simulink model "OFDM_Tx_HW"  (R2020a)
settings: Solver=FixedStepDiscrete  StartTime=0.0  StopTime=inf  RelTol=1e-3
InitFcn:
  | % Set parameters
  | fs = 20e6;
  | fclk = 240e6;
  | ssr = 2;
  | fdc = fclk*ssr*8;
  | 
  | % Load libraries
  | addpath('./lib');
  | 
  | % Load all required variables
  | load('variables/read_addr_data');
  | load('variables/read_addr_cp');
  | load('variables/read_addr_pream');
  | load('variables/read_addr_rx');
  | load('variables/pilot');
  | load('variables/sc_index');
  | load('variables/LTSfreq');
  | load('variables/STSfreq');
  | load('variables/LTSread');
  | load('variables/STSread');
  | 
  | run ./scripts/rfgen;
undefined symbols (not defined in the file): LTSfreq, LTSread, pilot, read_addr_cp, read_addr_data, read_addr_pream, STSfreq, STSread
libraries: hdlsllib x28, simulink x15, lib_rfsignalgenerator x1, dsphdlxfrm x1, dspsigops x1
settings Model: DataTypeOverride=Off  Creator=njb13206  LastModifiedBy=andy
settings OptimizationCC: BlockReduction=off  ConditionallyExecuteInputs=off  DefaultParameterBehavior=Inlined
settings DebuggingCC: AlgebraicLoopMsg=error  SingleTaskRateTransMsg=error  IntegerOverflowMsg=none  ParameterPrecisionLossMsg=none  IntegerSaturationMsg=none
settings HardwareCC: ProdBitPerPointer=32  ProdBitPerSizeT=32  ProdBitPerPtrDiffT=32  ProdLargestAtomicFloat=None  ProdIntDivRoundTo=Undefined  ProdEndianess=Unspecified  ProdWordSize=32  ProdHWDeviceType=ASIC/FPGA->ASIC/FPGA  TargetBitPerLong=64  TargetBitPerPointer=64  TargetBitPerSizeT=64  TargetBitPerPtrDiffT=64  TargetLongLongMode=on  TargetIntDivRoundTo=Zero  TargetEndianess=LittleEndian  TargetWordSize=64  TargetHWDeviceType=Custom Processor->MATLAB Host Computer  ProdEqTarget=off

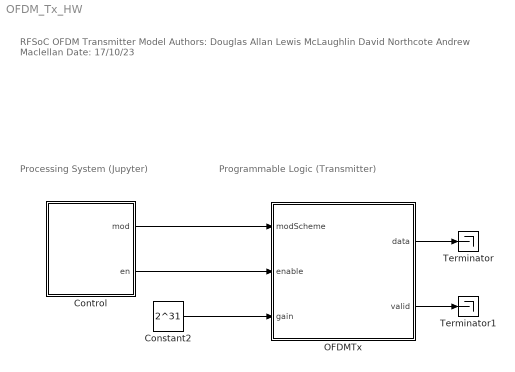
== system OFDM_Tx_HW ==
  note: RFSoC OFDM Transmitter Model
      | Authors: Douglas Allan
      | Lewis McLaughlin
      | David Northcote
      | Andrew Maclellan
      | Date: 17/10/23
  note: Programmable Logic (Transmitter)
  note: Processing System (Jupyter)
  Constant2 : Constant  Value=2^31  OutDataTypeStr=uint32  SampleTime=1/fclk
  Control : Subsystem  mask{mod_mask=128QAM, en=on}
      mask prompts: mod_mask "Modulation"; en "Enable"
      mask init:
      | % RF Signal Generator
      | if strcmpi(get_param(gcb, 'mod_mask'), 'BPSK')
      |     mod = 0;
      | elseif strcmpi(get_param(gcb, 'mod_mask'), 'QPSK')
      |     mod = 1;
      | elseif strcmpi(get_param(gcb, 'mod_mask'), '8PSK')
      |     mod = 2;
      | elseif strcmpi(get_param(gcb, 'mod_mask'), '16QAM')
      |     mod = 3;
      | elseif strcmpi(get_param(gcb, 'mod_mask'), '32QAM')
      |     mod = 4;
      | elseif strcmpi(get_param(gcb, 'mod_mask'), '64QAM')
      |     mod = 5;
      | elseif strcmpi(get_param(gcb, 'mod_mask'), '128QAM')
      |     mod = 6;
      | elseif strcmpi(get_param(gcb, 'mod_mask'), '256QAM')
      |     mod = 7;
      | elseif strcmpi(get_param(gcb, 'mod_mask'), '512QAM')
      |     mod = 8;
      | elseif strcmpi(get_param(gcb, 'mod_mask'), '1024QAM')
      |     mod = 9;
      | end
      mask TypeOptions mod_mask: BPSK | QPSK | 8PSK | 16QAM | 32QAM | 64QAM | 128QAM | 256QAM | 512QAM | 1024QAM
      mask DialogControl DescGroupVar Prompt: RF Signal Generator
      mask DialogControl DescTextVar Prompt: Exposes parameters the user can control from Jupyter when running on the target.
      mask DialogControl Container3 Prompt: Control
  OFDMTx : Subsystem  TreatAsAtomicUnit=on
  Terminator : Terminator
  Terminator1 : Terminator
  wires:
  Control/1(mod) -> OFDMTx/1(modScheme)
  Control/2(en) -> OFDMTx/2(enable)
  Constant2/1 -> OFDMTx/3(gain)
  OFDMTx/1(data) -> Terminator/1
  OFDMTx/2(valid) -> Terminator1/1

== system OFDM_Tx_HW/Control ==
  Constant2 : Constant  Value=en  OutDataTypeStr=boolean  SampleTime=1/(fclk)
  Constant7 : Constant  Value=mod  VectorParams1D=off  OutDataTypeStr=uint32  SampleTime=1/(fclk)
  Delay : Delay  DelayLength=randi(10)
  Delay3 : Delay  DelayLength=randi(10)
  mod : Outport  VectorParamsAs1DForOutWhenUnconnected=off
  en : Outport  Port=2  VectorParamsAs1DForOutWhenUnconnected=off
  wires:
  Constant2/1 -> Delay3/1
  Constant7/1 -> Delay/1
  Delay/1 -> mod/1
  Delay3/1 -> en/1

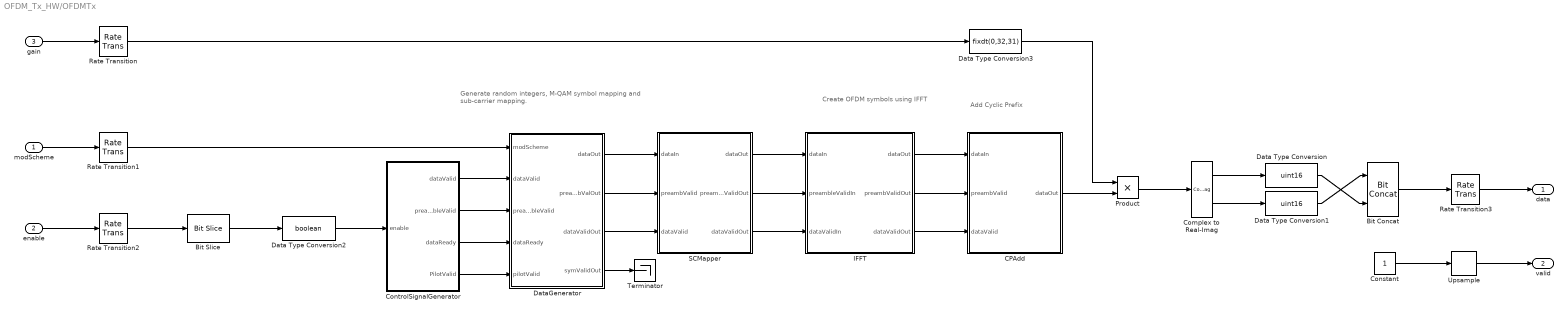
== system OFDM_Tx_HW/OFDMTx ==
  note: Generate random integers, M-QAM symbol mapping and sub-carrier
      | mapping.
  note: Add Cyclic Prefix
  note: Create OFDM symbols using
      | IFFT
  modScheme : Inport
  enable : Inport  Port=2
  gain : Inport  Port=3
  Bit Concat : hdlsllib/Logic and Bit Operations/Bit Concat  numInputs=2
  Bit Slice : hdlsllib/Logic and Bit Operations/Bit Slice  lidx=0  ridx=0
      settings: SourceProductBaseCode=SL
  CPAdd : Subsystem
  Complex to Real-Imag : ComplexToRealImag
  Constant : Constant  OutDataTypeStr=boolean  SampleTime=1/fs
  ControlSignalGenerator : Subsystem
  Data Type Conversion : DataTypeConversion  OutDataTypeStr=uint16  ConvertRealWorld=Stored Integer (SI)
  Data Type Conversion1 : DataTypeConversion  OutDataTypeStr=uint16  ConvertRealWorld=Stored Integer (SI)
  Data Type Conversion2 : DataTypeConversion  OutDataTypeStr=boolean  ConvertRealWorld=Stored Integer (SI)
  Data Type Conversion3 : DataTypeConversion  OutDataTypeStr=fixdt(0,32,31)  ConvertRealWorld=Stored Integer (SI)
  DataGenerator : Subsystem
  IFFT : Subsystem
  Product : Product  OutDataTypeStr=fixdt(1,16,14)  RndMeth=Round  SaturateOnIntegerOverflow=on
  Rate Transition : RateTransition  OutPortSampleTime=1/fs
  Rate Transition1 : RateTransition  OutPortSampleTime=1/fs
  Rate Transition2 : RateTransition  OutPortSampleTime=1/fs
  Rate Transition3 : RateTransition  OutPortSampleTime=1/fclk
  SCMapper : Subsystem
  Terminator : Terminator
  Upsample : dspsigops/Upsample  N=fclk/fs  phase=0  RateOptions=Allow multirate processing  ic=0  mode=Unused parameter value
  data : Outport  VectorParamsAs1DForOutWhenUnconnected=off
  valid : Outport  Port=2  VectorParamsAs1DForOutWhenUnconnected=off
  wires:
  Bit Slice/1 -> Data Type Conversion2/1
  enable/1 -> Rate Transition2/1
  Data Type Conversion/1 -> Bit Concat/2
  Data Type Conversion1/1 -> Bit Concat/1
  Complex to Real-Imag/2 -> Data Type Conversion1/1
  Complex to Real-Imag/1 -> Data Type Conversion/1
  modScheme/1 -> Rate Transition1/1
  DataGenerator/1(dataOut) -> SCMapper/1(dataIn)
  DataGenerator/2(preambValOut) -> SCMapper/2(preambValid)
  DataGenerator/3(dataValidOut) -> SCMapper/3(dataValid)
  SCMapper/1(dataOut) -> IFFT/1(dataIn)
  SCMapper/2(preambValidOut) -> IFFT/2(preambleValidIn)
  SCMapper/3(dataValidOut) -> IFFT/3("dataValidIn ")
  IFFT/1(dataOut) -> CPAdd/1(dataIn)
  IFFT/2(preambValidOut) -> CPAdd/2(preambValid)
  IFFT/3(dataValidOut) -> CPAdd/3(dataValid)
  ControlSignalGenerator/1(dataValid) -> DataGenerator/2(dataValid)
  ControlSignalGenerator/2(preambleValid) -> DataGenerator/3(preambleValid)
  Data Type Conversion2/1 -> ControlSignalGenerator/1(enable)
  DataGenerator/4(symValidOut) -> Terminator/1
  CPAdd/1(dataOut) -> Product/2
  Product/1 -> Complex to Real-Imag/1
  gain/1 -> Rate Transition/1
  Data Type Conversion3/1 -> Product/1
  Rate Transition/1 -> Data Type Conversion3/1
  Rate Transition1/1 -> DataGenerator/1(modScheme)
  Rate Transition2/1 -> Bit Slice/1
  Bit Concat/1 -> Rate Transition3/1
  Rate Transition3/1 -> data/1
  Constant/1 -> Upsample/1
  Upsample/1 -> valid/1
  ControlSignalGenerator/3(dataReady) -> DataGenerator/4(dataReady)
  ControlSignalGenerator/4(PilotValid) -> DataGenerator/5(pilotValid)

== system OFDM_Tx_HW/OFDMTx/CPAdd ==
  dataIn : Inport
  preambValid : Inport  Port=2
  dataValid : Inport  Port=3
  DataExtend : Subsystem
  LTFExtend : Subsystem
  Mux2 : MATLAB Function  TreatAsAtomicUnit=on
  STFExtend : Subsystem
  dataOut : Outport  VectorParamsAs1DForOutWhenUnconnected=off
  wires:
  preambValid/1 -> LTFExtend/2(preambVal), STFExtend/2(preambVal)
  dataIn/1 -> DataExtend/1(dataIn), LTFExtend/1(data), STFExtend/1(data)
  STFExtend/1(STFExtendOut) -> Mux2/1(sts)
  STFExtend/2(STFValidOut) -> Mux2/2(stsval)
  LTFExtend/1(LTFExtendOut) -> Mux2/3(lts)
  LTFExtend/2(LTFValidOut) -> Mux2/4(ltsval)
  DataExtend/1(dataOut) -> Mux2/5(data)
  DataExtend/2(dataValidOut) -> Mux2/6(dataval)
  Mux2/1(dataOut) -> dataOut/1
  dataValid/1 -> DataExtend/2(dataValid)

== system OFDM_Tx_HW/OFDMTx/ControlSignalGenerator ==
  enable : Inport
  Control Signal Generator : MATLAB Function  TreatAsAtomicUnit=on
  dataValid : Outport
  preambleValid : Outport  Port=2
  dataReady : Outport  Port=3
  PilotValid : Outport  Port=4
  wires:
  enable/1 -> Control Signal Generator/1(enable)  "enable"
  Control Signal Generator/1(preambleValid) -> preambleValid/1
  Control Signal Generator/2(dataValid) -> dataValid/1
  Control Signal Generator/3(dataReady) -> dataReady/1
  Control Signal Generator/4(pilotValid) -> PilotValid/1

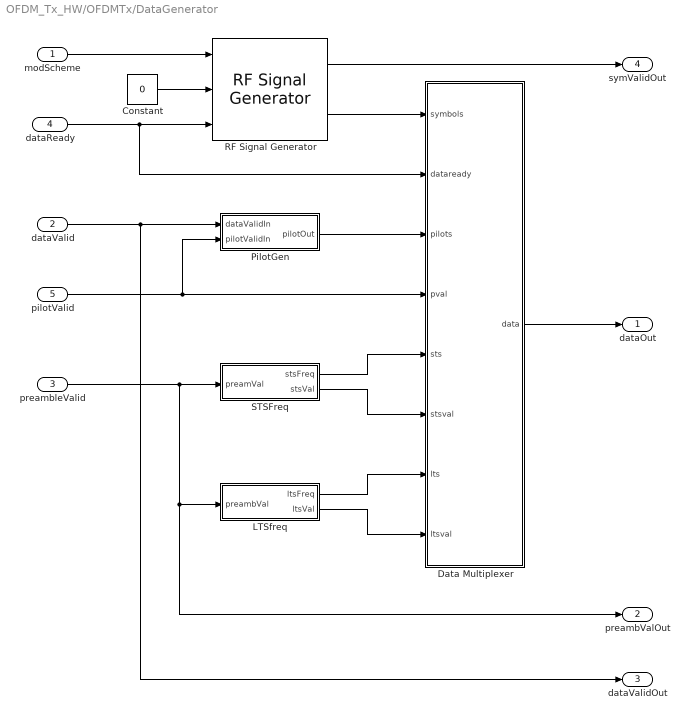
== system OFDM_Tx_HW/OFDMTx/DataGenerator ==
  modScheme : Inport
  dataValid : Inport  Port=2
  preambleValid : Inport  Port=3
  dataReady : Inport  Port=4
  pilotValid : Inport  Port=5
  Constant : Constant  Value=0  OutDataTypeStr=boolean  SampleTime=1/fs
  Data Multiplexer : MATLAB Function  TreatAsAtomicUnit=on
  LTSfreq : Subsystem
  PilotGen : Subsystem
  RF Signal Generator : lib_rfsignalgenerator/RF Signal Generator  SystemSampleTime=-1  Latency=0  AutoFrameSizeCalculation=off
  STSFreq : Subsystem
  dataOut : Outport  VectorParamsAs1DForOutWhenUnconnected=off
  preambValOut : Outport  Port=2  VectorParamsAs1DForOutWhenUnconnected=off
  dataValidOut : Outport  Port=3  VectorParamsAs1DForOutWhenUnconnected=off
  symValidOut : Outport  Port=4  VectorParamsAs1DForOutWhenUnconnected=off
  wires:
  dataValid/1 -> PilotGen/1(dataValidIn), dataValidOut/1
  preambleValid/1 -> STSFreq/1(preamVal), LTSfreq/1(preambVal), preambValOut/1
  LTSfreq/2(ltsVal) -> Data Multiplexer/8(ltsval)
  LTSfreq/1(ltsFreq) -> Data Multiplexer/7(lts)
  STSFreq/2(stsVal) -> Data Multiplexer/6(stsval)
  STSFreq/1(stsFreq) -> Data Multiplexer/5(sts)
  pilotValid/1 -> PilotGen/2(pilotValidIn), Data Multiplexer/4(pval)
  PilotGen/1(pilotOut) -> Data Multiplexer/3(pilots)
  RF Signal Generator/2 -> Data Multiplexer/1(symbols)
  Data Multiplexer/1(data) -> dataOut/1
  modScheme/1 -> RF Signal Generator/1
  RF Signal Generator/1 -> symValidOut/1
  Constant/1 -> RF Signal Generator/2
  dataReady/1 -> RF Signal Generator/3, Data Multiplexer/2(dataready)

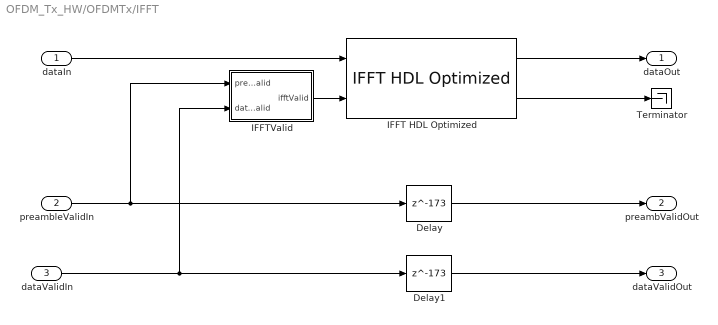
== system OFDM_Tx_HW/OFDMTx/IFFT ==
  dataIn : Inport
  preambleValidIn : Inport  Port=2
  "dataValidIn " : Inport  Port=3
  Delay : Delay  DelayLength=173  InitialCondition=0  UseCircularBuffer=on
  Delay1 : Delay  DelayLength=173  InitialCondition=0  UseCircularBuffer=on
  IFFT HDL Optimized : dsphdlxfrm/IFFT HDL Optimized  FFTLength=64  Architecture=Streaming Radix 2^2  ComplexMultiplication=Use 3 multipliers and 5 adders  BitReversedOutput=off  BitReversedInput=off  Normalize=on  SimulateUsing=Code generation  RoundingMethod=Floor  ResetInputPort=off  StartOutputPort=off  EndOutputPort=off
      settings: SourceProductBaseCode=DS
  IFFTValid : Subsystem
  Terminator : Terminator
  dataOut : Outport  VectorParamsAs1DForOutWhenUnconnected=off
  preambValidOut : Outport  Port=2  VectorParamsAs1DForOutWhenUnconnected=off
  dataValidOut : Outport  Port=3  VectorParamsAs1DForOutWhenUnconnected=off
  wires:
  dataIn/1 -> IFFT HDL Optimized/1
  IFFT HDL Optimized/2 -> Terminator/1
  "dataValidIn "/1 -> IFFTValid/2(dataValid), Delay1/1
  IFFTValid/1(ifftValid) -> IFFT HDL Optimized/2
  preambleValidIn/1 -> IFFTValid/1(preambleValid), Delay/1
  Delay/1 -> preambValidOut/1
  Delay1/1 -> dataValidOut/1
  IFFT HDL Optimized/1 -> dataOut/1

== system OFDM_Tx_HW/OFDMTx/SCMapper ==
  dataIn : Inport
  preambValid : Inport  Port=2
  dataValid : Inport  Port=3
  DataMapper : Subsystem
  Mux2 : MATLAB Function  TreatAsAtomicUnit=on
  PremableMapper : Subsystem
  dataOut : Outport  VectorParamsAs1DForOutWhenUnconnected=off
  preambValidOut : Outport  Port=2  VectorParamsAs1DForOutWhenUnconnected=off
  dataValidOut : Outport  Port=3  VectorParamsAs1DForOutWhenUnconnected=off
  wires:
  PremableMapper/1(preambleShiftOut) -> Mux2/1(preamb)
  PremableMapper/2(preambValOut) -> preambValidOut/1, Mux2/2(preambVal)
  DataMapper/1(dataOut) -> Mux2/3(data)
  DataMapper/2(dataValidOut) -> dataValidOut/1, Mux2/4(dataVal)
  dataIn/1 -> DataMapper/1(dataIn), PremableMapper/1(data)
  preambValid/1 -> PremableMapper/2(preambVal)
  dataValid/1 -> DataMapper/2(dataValid)
  Mux2/1(dataOut) -> dataOut/1

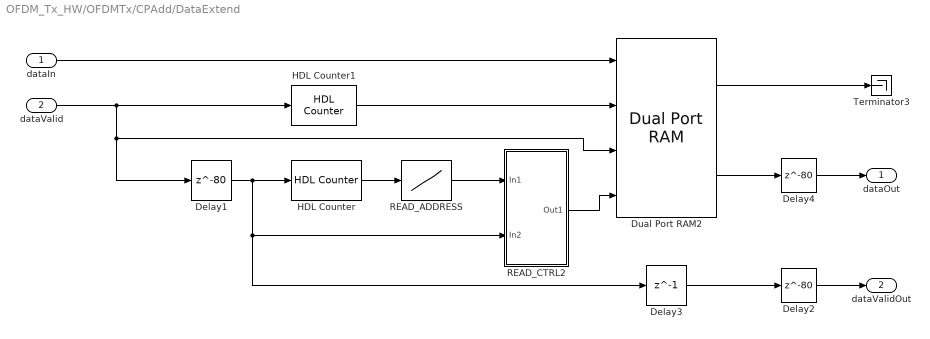
== system OFDM_Tx_HW/OFDMTx/CPAdd/DataExtend ==
  dataIn : Inport
  dataValid : Inport  Port=2
  Delay1 : Delay  DelayLength=80  InitialCondition=0  UseCircularBuffer=on
  Delay2 : Delay  DelayLength=80
  Delay3 : Delay  DelayLength=1  InitialCondition=0  UseCircularBuffer=on
  Delay4 : Delay  DelayLength=80
  Dual Port RAM2 : hdlsllib/HDL RAMs/Dual Port RAM  ram_size=8
      settings: SourceProductBaseCode=SL
  HDL Counter : hdlsllib/Sources/HDL Counter  CountType=Count limited  CountInit=0  CountStep=1  CountMax=159  CountFromType=Initial value  CountFrom=0  CountResetPort=off  CountLoadPort=off  CountEnbPort=on  CountDirPort=off  CountDataType=Unsigned  CountWordLen=8  CountFracLen=0  CountSampTime=1
  HDL Counter1 : hdlsllib/Sources/HDL Counter  CountType=Count limited  CountInit=0  CountStep=1  CountMax=159  CountFromType=Initial value  CountFrom=0  CountResetPort=off  CountLoadPort=off  CountEnbPort=on  CountDirPort=off  CountDataType=Unsigned  CountWordLen=8  CountFracLen=0  CountSampTime=1
  READ_ADDRESS : Lookup_n-D  NumberOfTableDimensions=1  LookupTableObject=''  BreakpointsForDimension1=[0:159]  BreakpointsForDimension1FirstPoint=10  BreakpointsForDimension2FirstPoint=10  BreakpointsForDimension1Spacing=12  BreakpointsForDimension2Spacing=12  IndexSearchMethod=Evenly spaced points  Table=read_addr_cp  TableDataTypeStr=fixdt(0,8,0)  InterpMethod=Flat  DiagnosticForOutOfRangeInput=Error  InternalRulePriority=Speed  OutDataTypeStr=fixdt(0,8,0)  RndMeth=Simplest  InputSameDT=on
  READ_CTRL2 : Subsystem
  Terminator3 : Terminator
  dataOut : Outport  VectorParamsAs1DForOutWhenUnconnected=off
  dataValidOut : Outport  Port=2  VectorParamsAs1DForOutWhenUnconnected=off
  wires:
  Delay4/1 -> dataOut/1
  Delay2/1 -> dataValidOut/1
  Dual Port RAM2/1 -> Terminator3/1
  READ_ADDRESS/1 -> READ_CTRL2/1(In1)
  HDL Counter/1 -> READ_ADDRESS/1
  dataIn/1 -> Dual Port RAM2/1
  HDL Counter1/1 -> Dual Port RAM2/2
  Delay1/1 -> HDL Counter/1, Delay3/1, READ_CTRL2/2(In2)
  Dual Port RAM2/2 -> Delay4/1
  dataValid/1 -> HDL Counter1/1, Dual Port RAM2/3, Delay1/1
  Delay3/1 -> Delay2/1
  READ_CTRL2/1(Out1) -> Dual Port RAM2/4

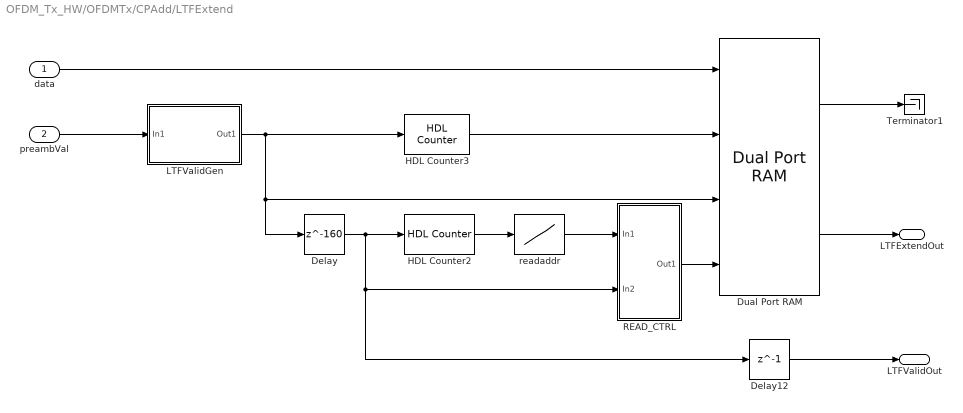
== system OFDM_Tx_HW/OFDMTx/CPAdd/LTFExtend ==
  data : Inport
  preambVal : Inport  Port=2
  Delay : Delay  DelayLength=160  InitialCondition=0  UseCircularBuffer=on
  Delay12 : Delay  DelayLength=1  InitialCondition=0  UseCircularBuffer=on
  Dual Port RAM : hdlsllib/HDL RAMs/Dual Port RAM  ram_size=8
      settings: SourceProductBaseCode=SL
  HDL Counter2 : hdlsllib/Sources/HDL Counter  CountType=Count limited  CountInit=0  CountStep=1  CountMax=159  CountFromType=Initial value  CountFrom=0  CountResetPort=off  CountLoadPort=off  CountEnbPort=on  CountDirPort=off  CountDataType=Unsigned  CountWordLen=8  CountFracLen=0  CountSampTime=1
  HDL Counter3 : hdlsllib/Sources/HDL Counter  CountType=Count limited  CountInit=0  CountStep=1  CountMax=159  CountFromType=Initial value  CountFrom=0  CountResetPort=off  CountLoadPort=off  CountEnbPort=on  CountDirPort=off  CountDataType=Unsigned  CountWordLen=8  CountFracLen=0  CountSampTime=1
  LTFValidGen : Subsystem
  READ_CTRL : Subsystem
  Terminator1 : Terminator
  readaddr : Lookup_n-D  NumberOfTableDimensions=1  LookupTableObject=''  BreakpointsForDimension1=0:159  BreakpointsForDimension1FirstPoint=10  BreakpointsForDimension2FirstPoint=10  BreakpointsForDimension1Spacing=12  BreakpointsForDimension2Spacing=12  IndexSearchMethod=Evenly spaced points  Table=LTSread  TableDataTypeStr=fixdt(0,8,0)  InterpMethod=Flat  DiagnosticForOutOfRangeInput=Error  InternalRulePriority=Speed  OutDataTypeStr=fixdt(0,8,0)  RndMeth=Simplest  InputSameDT=on
  LTFExtendOut : Outport  VectorParamsAs1DForOutWhenUnconnected=off
  LTFValidOut : Outport  Port=2  VectorParamsAs1DForOutWhenUnconnected=off
  wires:
  readaddr/1 -> READ_CTRL/1(In1)
  READ_CTRL/1(Out1) -> Dual Port RAM/4
  HDL Counter3/1 -> Dual Port RAM/2
  Delay/1 -> READ_CTRL/2(In2), Delay12/1, HDL Counter2/1
  Dual Port RAM/1 -> Terminator1/1
  Delay12/1 -> LTFValidOut/1
  HDL Counter2/1 -> readaddr/1
  data/1 -> Dual Port RAM/1
  Dual Port RAM/2 -> LTFExtendOut/1
  preambVal/1 -> LTFValidGen/1(In1)
  LTFValidGen/1(Out1) -> Dual Port RAM/3, Delay/1, HDL Counter3/1

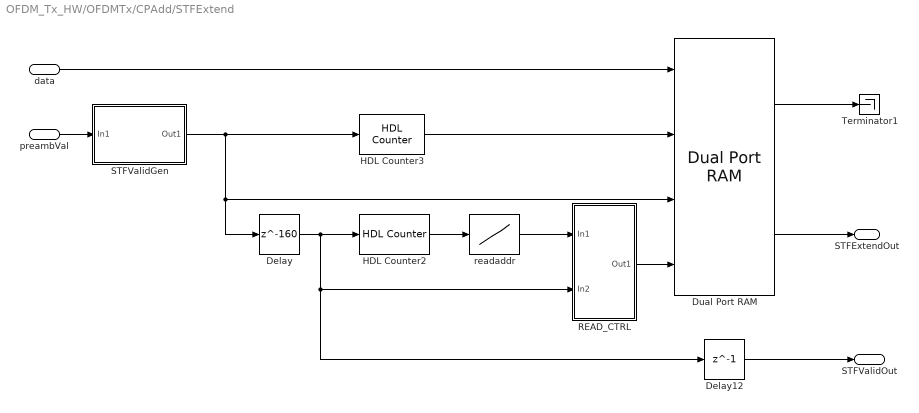
== system OFDM_Tx_HW/OFDMTx/CPAdd/STFExtend ==
  data : Inport
  preambVal : Inport  Port=2
  Delay : Delay  DelayLength=160  InitialCondition=0  UseCircularBuffer=on
  Delay12 : Delay  DelayLength=1  InitialCondition=0  UseCircularBuffer=on
  Dual Port RAM : hdlsllib/HDL RAMs/Dual Port RAM  ram_size=8
      settings: SourceProductBaseCode=SL
  HDL Counter2 : hdlsllib/Sources/HDL Counter  CountType=Count limited  CountInit=0  CountStep=1  CountMax=159  CountFromType=Initial value  CountFrom=0  CountResetPort=off  CountLoadPort=off  CountEnbPort=on  CountDirPort=off  CountDataType=Unsigned  CountWordLen=8  CountFracLen=0  CountSampTime=1
  HDL Counter3 : hdlsllib/Sources/HDL Counter  CountType=Count limited  CountInit=0  CountStep=1  CountMax=159  CountFromType=Initial value  CountFrom=0  CountResetPort=off  CountLoadPort=off  CountEnbPort=on  CountDirPort=off  CountDataType=Unsigned  CountWordLen=8  CountFracLen=0  CountSampTime=1
  READ_CTRL : Subsystem
  STFValidGen : Subsystem
  Terminator1 : Terminator
  readaddr : Lookup_n-D  NumberOfTableDimensions=1  LookupTableObject=''  BreakpointsForDimension1=0:159  BreakpointsForDimension1FirstPoint=10  BreakpointsForDimension2FirstPoint=10  BreakpointsForDimension1Spacing=12  BreakpointsForDimension2Spacing=12  IndexSearchMethod=Evenly spaced points  Table=STSread  TableDataTypeStr=fixdt(0,8,0)  InterpMethod=Flat  DiagnosticForOutOfRangeInput=Error  InternalRulePriority=Speed  OutDataTypeStr=fixdt(0,8,0)  RndMeth=Simplest  InputSameDT=on
  STFExtendOut : Outport  VectorParamsAs1DForOutWhenUnconnected=off
  STFValidOut : Outport  Port=2  VectorParamsAs1DForOutWhenUnconnected=off
  wires:
  Dual Port RAM/2 -> STFExtendOut/1
  data/1 -> Dual Port RAM/1
  HDL Counter2/1 -> readaddr/1
  Delay12/1 -> STFValidOut/1
  Dual Port RAM/1 -> Terminator1/1
  Delay/1 -> HDL Counter2/1, Delay12/1, READ_CTRL/2(In2)
  HDL Counter3/1 -> Dual Port RAM/2
  READ_CTRL/1(Out1) -> Dual Port RAM/4
  preambVal/1 -> STFValidGen/1(In1)
  readaddr/1 -> READ_CTRL/1(In1)
  STFValidGen/1(Out1) -> HDL Counter3/1, Dual Port RAM/3, Delay/1

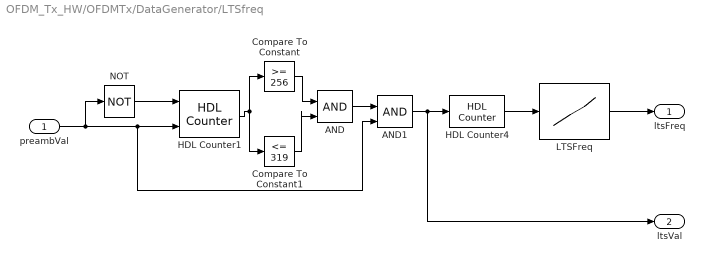
== system OFDM_Tx_HW/OFDMTx/DataGenerator/LTSfreq ==
  preambVal : Inport
  AND : Logic  IconShape=distinctive  AllPortsSameDT=off  OutDataTypeStr=boolean
  AND1 : Logic  IconShape=distinctive  AllPortsSameDT=off  OutDataTypeStr=boolean
  Compare To Constant : simulink/Logic and Bit Operations/Compare To Constant  relop=>=  const=256  OutDataTypeStr=boolean
  Compare To Constant1 : simulink/Logic and Bit Operations/Compare To Constant  relop=<=  const=319  OutDataTypeStr=boolean
  HDL Counter1 : hdlsllib/Sources/HDL Counter  CountType=Count limited  CountInit=0  CountStep=1  CountMax=319  CountFromType=Initial value  CountFrom=0  CountResetPort=on  CountLoadPort=off  CountEnbPort=on  CountDirPort=off  CountDataType=Unsigned  CountWordLen=9  CountFracLen=0  CountSampTime=1
  HDL Counter4 : hdlsllib/Sources/HDL Counter  CountType=Count limited  CountInit=0  CountStep=1  CountMax=63  CountFromType=Initial value  CountFrom=0  CountResetPort=off  CountLoadPort=off  CountEnbPort=on  CountDirPort=off  CountDataType=Unsigned  CountWordLen=6  CountFracLen=0  CountSampTime=1
  LTSFreq : Lookup_n-D  NumberOfTableDimensions=1  LookupTableObject=''  BreakpointsForDimension1=0:63  BreakpointsForDimension1FirstPoint=10  BreakpointsForDimension2FirstPoint=10  BreakpointsForDimension1Spacing=12  BreakpointsForDimension2Spacing=12  IndexSearchMethod=Evenly spaced points  Table=LTSfreq  TableDataTypeStr=fixdt(1,16,14)  InterpMethod=Flat  DiagnosticForOutOfRangeInput=Error  InternalRulePriority=Speed  OutDataTypeStr=fixdt(1,16,14)  RndMeth=Simplest  InputSameDT=on
  NOT : Logic  Operator=NOT  IconShape=distinctive  AllPortsSameDT=off  OutDataTypeStr=boolean
  ltsFreq : Outport  VectorParamsAs1DForOutWhenUnconnected=off
  ltsVal : Outport  Port=2  VectorParamsAs1DForOutWhenUnconnected=off
  wires:
  HDL Counter4/1 -> LTSFreq/1
  Compare To Constant/1 -> AND/1
  HDL Counter1/1 -> Compare To Constant1/1, Compare To Constant/1
  Compare To Constant1/1 -> AND/2
  NOT/1 -> HDL Counter1/1
  AND/1 -> AND1/1
  preambVal/1 -> NOT/1, AND1/2, HDL Counter1/2
  AND1/1 -> ltsVal/1, HDL Counter4/1
  LTSFreq/1 -> ltsFreq/1

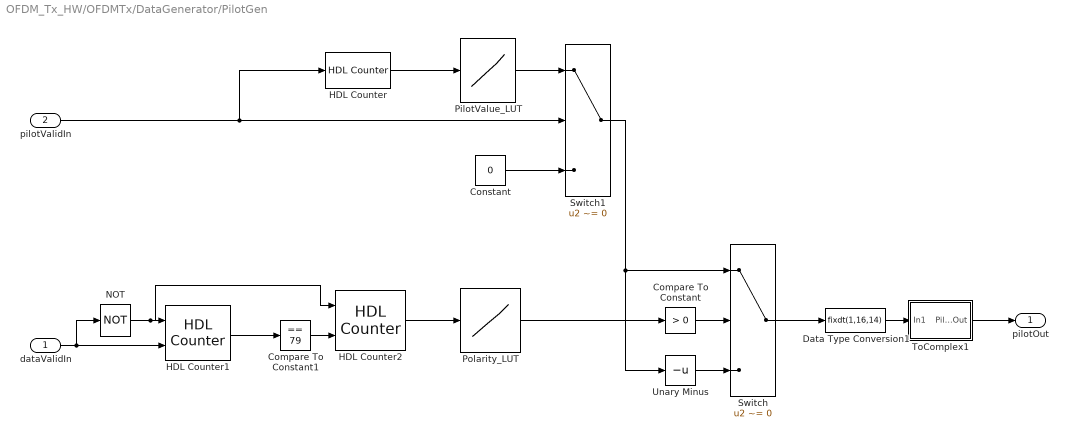
== system OFDM_Tx_HW/OFDMTx/DataGenerator/PilotGen ==
  dataValidIn : Inport
  pilotValidIn : Inport  Port=2
  Compare To Constant : simulink/Logic and Bit Operations/Compare To Constant  relop=>  const=0  OutDataTypeStr=boolean
  Compare To Constant1 : simulink/Logic and Bit Operations/Compare To Constant  relop===  const=79  OutDataTypeStr=boolean
  Constant : Constant  Value=0  OutDataTypeStr=fixdt(1,2,0)  SampleTime=1/fs
  Data Type Conversion1 : DataTypeConversion  OutDataTypeStr=fixdt(1,16,14)
  HDL Counter : hdlsllib/Sources/HDL Counter  CountType=Count limited  CountInit=0  CountStep=1  CountMax=3  CountFromType=Initial value  CountFrom=0  CountResetPort=off  CountLoadPort=off  CountEnbPort=on  CountDirPort=off  CountDataType=Unsigned  CountWordLen=2  CountFracLen=0  CountSampTime=1
  HDL Counter1 : hdlsllib/Sources/HDL Counter  CountType=Count limited  CountInit=0  CountStep=1  CountMax=79  CountFromType=Initial value  CountFrom=0  CountResetPort=on  CountLoadPort=off  CountEnbPort=on  CountDirPort=off  CountDataType=Unsigned  CountWordLen=8  CountFracLen=0  CountSampTime=1
  HDL Counter2 : hdlsllib/Sources/HDL Counter  CountType=Count limited  CountInit=0  CountStep=1  CountMax=126  CountFromType=Initial value  CountFrom=0  CountResetPort=on  CountLoadPort=off  CountEnbPort=on  CountDirPort=off  CountDataType=Unsigned  CountWordLen=7  CountFracLen=0  CountSampTime=1
  NOT : Logic  Operator=NOT  IconShape=distinctive  AllPortsSameDT=off  OutDataTypeStr=boolean
  PilotValue_LUT : Lookup_n-D  NumberOfTableDimensions=1  LookupTableObject=''  BreakpointsForDimension1=[0:3]  BreakpointsForDimension1FirstPoint=10  BreakpointsForDimension2FirstPoint=10  BreakpointsForDimension1Spacing=12  BreakpointsForDimension2Spacing=12  IndexSearchMethod=Evenly spaced points  Table=[1 1 1 -1]  TableDataTypeStr=fixdt(1,2,0)  InterpMethod=Flat  DiagnosticForOutOfRangeInput=Error  InternalRulePriority=Speed  OutDataTypeStr=fixdt(1,2,0)  RndMeth=Simplest  InputSameDT=on
  Polarity_LUT : Lookup_n-D  NumberOfTableDimensions=1  LookupTableObject=''  BreakpointsForDimension1=[0:126]  BreakpointsForDimension1FirstPoint=10  BreakpointsForDimension2FirstPoint=10  BreakpointsForDimension1Spacing=12  BreakpointsForDimension2Spacing=12  IndexSearchMethod=Evenly spaced points  Table=pilot  TableDataTypeStr=fixdt(1,2,0)  InterpMethod=Flat  DiagnosticForOutOfRangeInput=Error  InternalRulePriority=Speed  OutDataTypeStr=fixdt(1,2,0)  RndMeth=Simplest  InputSameDT=on
  Switch : Switch  Criteria=u2 ~= 0
  Switch1 : Switch  Criteria=u2 ~= 0
  ToComplex1 : Subsystem
  Unary Minus : UnaryMinus
  pilotOut : Outport  VectorParamsAs1DForOutWhenUnconnected=off
  wires:
  HDL Counter/1 -> PilotValue_LUT/1
  Data Type Conversion1/1 -> ToComplex1/1(In1)
  dataValidIn/1 -> HDL Counter1/2, NOT/1
  HDL Counter1/1 -> Compare To Constant1/1
  NOT/1 -> HDL Counter2/1, HDL Counter1/1
  Compare To Constant1/1 -> HDL Counter2/2
  HDL Counter2/1 -> Polarity_LUT/1
  ToComplex1/1(PilotOut) -> pilotOut/1
  pilotValidIn/1 -> HDL Counter/1, Switch1/2
  Polarity_LUT/1 -> Compare To Constant/1
  Compare To Constant/1 -> Switch/2
  Unary Minus/1 -> Switch/3
  Switch/1 -> Data Type Conversion1/1
  PilotValue_LUT/1 -> Switch1/1
  Switch1/1 -> Unary Minus/1, Switch/1
  Constant/1 -> Switch1/3

== system OFDM_Tx_HW/OFDMTx/DataGenerator/STSFreq ==
  preamVal : Inport
  AND : Logic  IconShape=distinctive  AllPortsSameDT=off  OutDataTypeStr=boolean
  AND1 : Logic  IconShape=distinctive  AllPortsSameDT=off  OutDataTypeStr=boolean
  Compare To Constant : simulink/Logic and Bit Operations/Compare To Constant  relop=>=  const=96  OutDataTypeStr=boolean
  Compare To Constant1 : simulink/Logic and Bit Operations/Compare To Constant  relop=<=  const=159  OutDataTypeStr=boolean
  HDL Counter : hdlsllib/Sources/HDL Counter  CountType=Count limited  CountInit=0  CountStep=1  CountMax=63  CountFromType=Initial value  CountFrom=0  CountResetPort=off  CountLoadPort=off  CountEnbPort=on  CountDirPort=off  CountDataType=Unsigned  CountWordLen=6  CountFracLen=0  CountSampTime=1
  HDL Counter1 : hdlsllib/Sources/HDL Counter  CountType=Count limited  CountInit=0  CountStep=1  CountMax=319  CountFromType=Initial value  CountFrom=0  CountResetPort=on  CountLoadPort=off  CountEnbPort=on  CountDirPort=off  CountDataType=Unsigned  CountWordLen=9  CountFracLen=0  CountSampTime=1
  NOT : Logic  Operator=NOT  IconShape=distinctive  AllPortsSameDT=off  OutDataTypeStr=boolean
  STSFreq : Lookup_n-D  NumberOfTableDimensions=1  LookupTableObject=''  BreakpointsForDimension1=[0:63]  BreakpointsForDimension1FirstPoint=10  BreakpointsForDimension2FirstPoint=10  BreakpointsForDimension1Spacing=12  BreakpointsForDimension2Spacing=12  IndexSearchMethod=Evenly spaced points  Table=STSfreq  TableDataTypeStr=fixdt(1,16,14)  InterpMethod=Flat  DiagnosticForOutOfRangeInput=Error  InternalRulePriority=Speed  OutDataTypeStr=fixdt(1,16,14)  RndMeth=Simplest  InputSameDT=on
  stsFreq : Outport  VectorParamsAs1DForOutWhenUnconnected=off
  stsVal : Outport  Port=2  VectorParamsAs1DForOutWhenUnconnected=off
  wires:
  HDL Counter/1 -> STSFreq/1
  AND/1 -> AND1/1
  HDL Counter1/1 -> Compare To Constant1/1, Compare To Constant/1
  NOT/1 -> HDL Counter1/1
  Compare To Constant/1 -> AND/1
  Compare To Constant1/1 -> AND/2
  preamVal/1 -> NOT/1, AND1/2, HDL Counter1/2
  AND1/1 -> stsVal/1, HDL Counter/1
  STSFreq/1 -> stsFreq/1

== system OFDM_Tx_HW/OFDMTx/IFFT/IFFTValid ==
  preambleValid : Inport
  dataValid : Inport  Port=2
  Switch : Switch  Criteria=u2 ~= 0
  dataIFFTValid : Subsystem
  preambIFFTValid : Subsystem
  ifftValid : Outport  VectorParamsAs1DForOutWhenUnconnected=off
  wires:
  preambleValid/1 -> Switch/2, preambIFFTValid/1(preambValid)
  preambIFFTValid/1(preambIFFTValidOut) -> Switch/1
  dataValid/1 -> dataIFFTValid/1(dataValidIn)
  dataIFFTValid/1(dataIFFTValidOut) -> Switch/3
  Switch/1 -> ifftValid/1

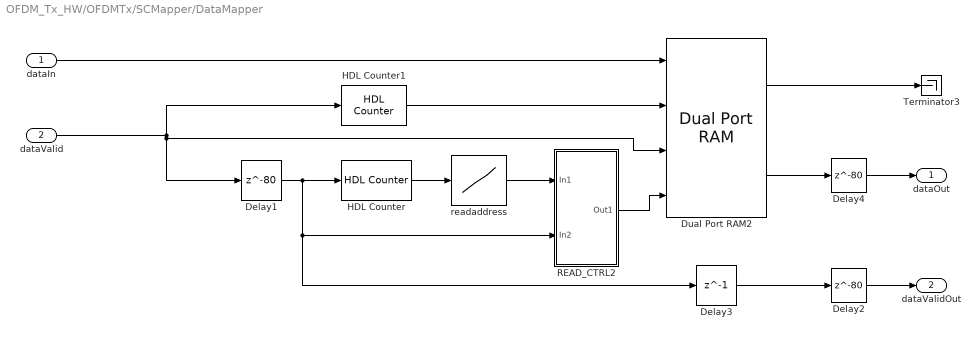
== system OFDM_Tx_HW/OFDMTx/SCMapper/DataMapper ==
  dataIn : Inport
  dataValid : Inport  Port=2
  Delay1 : Delay  DelayLength=80  InitialCondition=0  UseCircularBuffer=on
  Delay2 : Delay  DelayLength=80
  Delay3 : Delay  DelayLength=1  InitialCondition=0  UseCircularBuffer=on
  Delay4 : Delay  DelayLength=80
  Dual Port RAM2 : hdlsllib/HDL RAMs/Dual Port RAM  ram_size=8
      settings: SourceProductBaseCode=SL
  HDL Counter : hdlsllib/Sources/HDL Counter  CountType=Count limited  CountInit=0  CountStep=1  CountMax=159  CountFromType=Initial value  CountFrom=0  CountResetPort=off  CountLoadPort=off  CountEnbPort=on  CountDirPort=off  CountDataType=Unsigned  CountWordLen=8  CountFracLen=0  CountSampTime=1
  HDL Counter1 : hdlsllib/Sources/HDL Counter  CountType=Count limited  CountInit=0  CountStep=1  CountMax=159  CountFromType=Initial value  CountFrom=0  CountResetPort=off  CountLoadPort=off  CountEnbPort=on  CountDirPort=off  CountDataType=Unsigned  CountWordLen=8  CountFracLen=0  CountSampTime=1
  READ_CTRL2 : Subsystem
  Terminator3 : Terminator
  readaddress : Lookup_n-D  NumberOfTableDimensions=1  LookupTableObject=''  BreakpointsForDimension1=[0:159]  BreakpointsForDimension1FirstPoint=10  BreakpointsForDimension2FirstPoint=10  BreakpointsForDimension1Spacing=12  BreakpointsForDimension2Spacing=12  IndexSearchMethod=Evenly spaced points  Table=read_addr_data  TableDataTypeStr=fixdt(0,8,0)  InterpMethod=Flat  DiagnosticForOutOfRangeInput=Error  InternalRulePriority=Speed  OutDataTypeStr=fixdt(0,8,0)  RndMeth=Simplest  InputSameDT=on
  dataOut : Outport  VectorParamsAs1DForOutWhenUnconnected=off
  dataValidOut : Outport  Port=2  VectorParamsAs1DForOutWhenUnconnected=off
  wires:
  READ_CTRL2/1(Out1) -> Dual Port RAM2/4
  Delay3/1 -> Delay2/1
  dataValid/1 -> HDL Counter1/1, Delay1/1, Dual Port RAM2/3
  Dual Port RAM2/2 -> Delay4/1
  Delay1/1 -> READ_CTRL2/2(In2), Delay3/1, HDL Counter/1
  HDL Counter1/1 -> Dual Port RAM2/2
  dataIn/1 -> Dual Port RAM2/1
  HDL Counter/1 -> readaddress/1
  readaddress/1 -> READ_CTRL2/1(In1)
  Dual Port RAM2/1 -> Terminator3/1
  Delay2/1 -> dataValidOut/1
  Delay4/1 -> dataOut/1

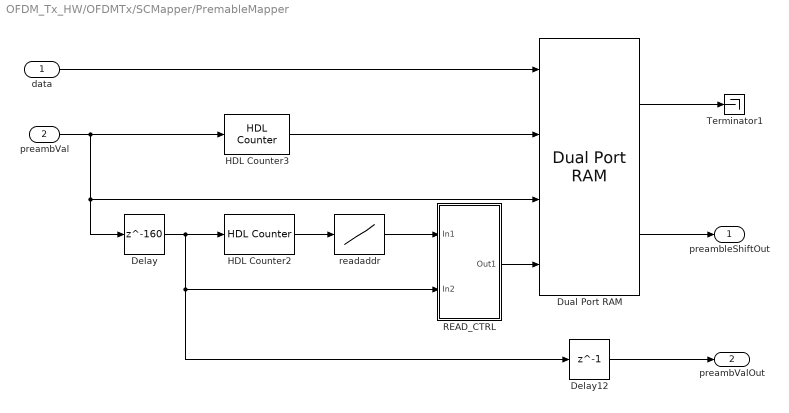
== system OFDM_Tx_HW/OFDMTx/SCMapper/PremableMapper ==
  data : Inport
  preambVal : Inport  Port=2
  Delay : Delay  DelayLength=160  InitialCondition=0  UseCircularBuffer=on
  Delay12 : Delay  DelayLength=1  InitialCondition=0  UseCircularBuffer=on
  Dual Port RAM : hdlsllib/HDL RAMs/Dual Port RAM  ram_size=9
      settings: SourceProductBaseCode=SL
  HDL Counter2 : hdlsllib/Sources/HDL Counter  CountType=Count limited  CountInit=0  CountStep=1  CountMax=319  CountFromType=Initial value  CountFrom=0  CountResetPort=off  CountLoadPort=off  CountEnbPort=on  CountDirPort=off  CountDataType=Unsigned  CountWordLen=9  CountFracLen=0  CountSampTime=1
  HDL Counter3 : hdlsllib/Sources/HDL Counter  CountType=Count limited  CountInit=0  CountStep=1  CountMax=319  CountFromType=Initial value  CountFrom=0  CountResetPort=off  CountLoadPort=off  CountEnbPort=on  CountDirPort=off  CountDataType=Unsigned  CountWordLen=9  CountFracLen=0  CountSampTime=1
  READ_CTRL : Subsystem
  Terminator1 : Terminator
  readaddr : Lookup_n-D  NumberOfTableDimensions=1  LookupTableObject=''  BreakpointsForDimension1=0:319  BreakpointsForDimension1FirstPoint=10  BreakpointsForDimension2FirstPoint=10  BreakpointsForDimension1Spacing=12  BreakpointsForDimension2Spacing=12  IndexSearchMethod=Evenly spaced points  Table=read_addr_pream  TableDataTypeStr=fixdt(0,9,0)  InterpMethod=Flat  DiagnosticForOutOfRangeInput=Error  InternalRulePriority=Speed  OutDataTypeStr=fixdt(0,9,0)  RndMeth=Simplest  InputSameDT=on
  preambleShiftOut : Outport  VectorParamsAs1DForOutWhenUnconnected=off
  preambValOut : Outport  Port=2  VectorParamsAs1DForOutWhenUnconnected=off
  wires:
  readaddr/1 -> READ_CTRL/1(In1)
  preambVal/1 -> Delay/1, Dual Port RAM/3, HDL Counter3/1
  READ_CTRL/1(Out1) -> Dual Port RAM/4
  HDL Counter3/1 -> Dual Port RAM/2
  Delay/1 -> READ_CTRL/2(In2), Delay12/1, HDL Counter2/1
  Dual Port RAM/1 -> Terminator1/1
  Delay12/1 -> preambValOut/1
  HDL Counter2/1 -> readaddr/1
  data/1 -> Dual Port RAM/1
  Dual Port RAM/2 -> preambleShiftOut/1

== system OFDM_Tx_HW/OFDMTx/CPAdd/DataExtend/READ_CTRL2 ==
  In1 : Inport
  In2 : Inport  Port=2
  Constant : Constant  Value=0  OutDataTypeStr=fixdt(0,8,0)  SampleTime=1/fs
  Switch : Switch  Criteria=u2 ~= 0
  Out1 : Outport  VectorParamsAs1DForOutWhenUnconnected=off
  wires:
  Constant/1 -> Switch/3
  In2/1 -> Switch/2
  In1/1 -> Switch/1
  Switch/1 -> Out1/1

== system OFDM_Tx_HW/OFDMTx/CPAdd/LTFExtend/LTFValidGen ==
  In1 : Inport
  AND : Logic  IconShape=distinctive  AllPortsSameDT=off  OutDataTypeStr=boolean
  AND1 : Logic  IconShape=distinctive  AllPortsSameDT=off  OutDataTypeStr=boolean
  Compare To Constant : simulink/Logic and Bit Operations/Compare To Constant  relop=>=  const=160  OutDataTypeStr=boolean
  Compare To Constant1 : simulink/Logic and Bit Operations/Compare To Constant  relop=<=  const=319  OutDataTypeStr=boolean
  HDL Counter : hdlsllib/Sources/HDL Counter  CountType=Count limited  CountInit=0  CountStep=1  CountMax=319  CountFromType=Initial value  CountFrom=0  CountResetPort=on  CountLoadPort=off  CountEnbPort=on  CountDirPort=off  CountDataType=Unsigned  CountWordLen=9  CountFracLen=0  CountSampTime=1
  NOT : Logic  Operator=NOT  IconShape=distinctive  AllPortsSameDT=off  OutDataTypeStr=boolean
  Out1 : Outport  VectorParamsAs1DForOutWhenUnconnected=off
  wires:
  Compare To Constant/1 -> AND/1
  In1/1 -> NOT/1, AND1/2, HDL Counter/2
  HDL Counter/1 -> Compare To Constant1/1, Compare To Constant/1
  Compare To Constant1/1 -> AND/2
  AND1/1 -> Out1/1
  AND/1 -> AND1/1
  NOT/1 -> HDL Counter/1

== system OFDM_Tx_HW/OFDMTx/CPAdd/LTFExtend/READ_CTRL ==
  In1 : Inport
  In2 : Inport  Port=2
  Constant : Constant  Value=0  OutDataTypeStr=fixdt(0,8,0)  SampleTime=1/fs
  Switch : Switch  Criteria=u2 ~= 0
  Out1 : Outport  VectorParamsAs1DForOutWhenUnconnected=off
  wires:
  Switch/1 -> Out1/1
  In1/1 -> Switch/1
  In2/1 -> Switch/2
  Constant/1 -> Switch/3

== system OFDM_Tx_HW/OFDMTx/CPAdd/STFExtend/READ_CTRL ==
  In1 : Inport
  In2 : Inport  Port=2
  Constant : Constant  Value=0  OutDataTypeStr=fixdt(0,8,0)  SampleTime=1/fs
  Switch : Switch  Criteria=u2 ~= 0
  Out1 : Outport  VectorParamsAs1DForOutWhenUnconnected=off
  wires:
  Constant/1 -> Switch/3
  In2/1 -> Switch/2
  In1/1 -> Switch/1
  Switch/1 -> Out1/1

== system OFDM_Tx_HW/OFDMTx/CPAdd/STFExtend/STFValidGen ==
  In1 : Inport
  AND : Logic  IconShape=distinctive  AllPortsSameDT=off  OutDataTypeStr=boolean
  AND1 : Logic  IconShape=distinctive  AllPortsSameDT=off  OutDataTypeStr=boolean
  Compare To Constant : simulink/Logic and Bit Operations/Compare To Constant  relop=>=  const=0  OutDataTypeStr=boolean
  Compare To Constant1 : simulink/Logic and Bit Operations/Compare To Constant  relop=<=  const=159  OutDataTypeStr=boolean
  HDL Counter : hdlsllib/Sources/HDL Counter  CountType=Count limited  CountInit=0  CountStep=1  CountMax=319  CountFromType=Initial value  CountFrom=0  CountResetPort=on  CountLoadPort=off  CountEnbPort=on  CountDirPort=off  CountDataType=Unsigned  CountWordLen=9  CountFracLen=0  CountSampTime=1
  NOT : Logic  Operator=NOT  IconShape=distinctive  AllPortsSameDT=off  OutDataTypeStr=boolean
  Out1 : Outport  VectorParamsAs1DForOutWhenUnconnected=off
  wires:
  Compare To Constant/1 -> AND/1
  In1/1 -> NOT/1, AND1/2, HDL Counter/2
  HDL Counter/1 -> Compare To Constant1/1, Compare To Constant/1
  Compare To Constant1/1 -> AND/2
  AND1/1 -> Out1/1
  AND/1 -> AND1/1
  NOT/1 -> HDL Counter/1

== system OFDM_Tx_HW/OFDMTx/DataGenerator/PilotGen/ToComplex1 ==
  In1 : Inport
  Constant1 : Constant  Value=0  OutDataTypeStr=fixdt(1,16,14)  SampleTime=1/fs
  Real-Imag to Complex : RealImagToComplex
  PilotOut : Outport  VectorParamsAs1DForOutWhenUnconnected=off
  wires:
  Constant1/1 -> Real-Imag to Complex/2
  In1/1 -> Real-Imag to Complex/1
  Real-Imag to Complex/1 -> PilotOut/1

== system OFDM_Tx_HW/OFDMTx/IFFT/IFFTValid/dataIFFTValid ==
  dataValidIn : Inport
  Compare To Constant : simulink/Logic and Bit Operations/Compare To Constant  relop=>=  const=17  OutDataTypeStr=boolean
  Logical Operator : Logic  Operator=NOT  IconShape=distinctive  AllPortsSameDT=off  OutDataTypeStr=boolean
  SAMPLE_COUNTER : hdlsllib/Sources/HDL Counter  CountType=Count limited  CountInit=1  CountStep=1  CountMax=80  CountFromType=Initial value  CountFrom=1  CountResetPort=on  CountLoadPort=off  CountEnbPort=on  CountDirPort=off  CountDataType=Unsigned  CountWordLen=7  CountFracLen=0  CountSampTime=1
  dataIFFTValidOut : Outport  VectorParamsAs1DForOutWhenUnconnected=off
  wires:
  dataValidIn/1 -> SAMPLE_COUNTER/2, Logical Operator/1
  Compare To Constant/1 -> dataIFFTValidOut/1
  Logical Operator/1 -> SAMPLE_COUNTER/1
  SAMPLE_COUNTER/1 -> Compare To Constant/1

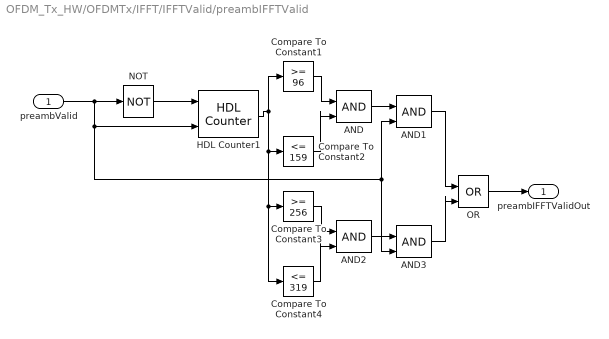
== system OFDM_Tx_HW/OFDMTx/IFFT/IFFTValid/preambIFFTValid ==
  preambValid : Inport
  AND{,1..3} (4 alike) : Logic  IconShape=distinctive  AllPortsSameDT=off  OutDataTypeStr=boolean
  Compare To Constant1 : simulink/Logic and Bit Operations/Compare To Constant  relop=>=  const=96  OutDataTypeStr=boolean
  Compare To Constant2 : simulink/Logic and Bit Operations/Compare To Constant  relop=<=  const=159  OutDataTypeStr=boolean
  Compare To Constant3 : simulink/Logic and Bit Operations/Compare To Constant  relop=>=  const=256  OutDataTypeStr=boolean
  Compare To Constant4 : simulink/Logic and Bit Operations/Compare To Constant  relop=<=  const=319  OutDataTypeStr=boolean
  HDL Counter1 : hdlsllib/Sources/HDL Counter  CountType=Count limited  CountInit=0  CountStep=1  CountMax=319  CountFromType=Initial value  CountFrom=0  CountResetPort=on  CountLoadPort=off  CountEnbPort=on  CountDirPort=off  CountDataType=Unsigned  CountWordLen=9  CountFracLen=0  CountSampTime=1
  NOT : Logic  Operator=NOT  IconShape=distinctive  AllPortsSameDT=off  OutDataTypeStr=boolean
  OR : Logic  Operator=OR  IconShape=distinctive  AllPortsSameDT=off  OutDataTypeStr=boolean
  preambIFFTValidOut : Outport  VectorParamsAs1DForOutWhenUnconnected=off
  wires:
  AND/1 -> AND1/1
  AND2/1 -> AND3/1
  HDL Counter1/1 -> Compare To Constant4/1, Compare To Constant3/1, Compare To Constant2/1, Compare To Constant1/1
  OR/1 -> preambIFFTValidOut/1
  preambValid/1 -> HDL Counter1/2, AND3/2, AND1/2, NOT/1
  Compare To Constant1/1 -> AND/1
  Compare To Constant4/1 -> AND2/2
  AND1/1 -> OR/1
  AND3/1 -> OR/2
  Compare To Constant2/1 -> AND/2
  NOT/1 -> HDL Counter1/1
  Compare To Constant3/1 -> AND2/1

== system OFDM_Tx_HW/OFDMTx/SCMapper/DataMapper/READ_CTRL2 ==
  In1 : Inport
  In2 : Inport  Port=2
  Constant : Constant  Value=0  OutDataTypeStr=fixdt(0,8,0)  SampleTime=1/fs
  Switch : Switch  Criteria=u2 ~= 0
  Out1 : Outport  VectorParamsAs1DForOutWhenUnconnected=off
  wires:
  Switch/1 -> Out1/1
  In1/1 -> Switch/1
  In2/1 -> Switch/2
  Constant/1 -> Switch/3

== system OFDM_Tx_HW/OFDMTx/SCMapper/PremableMapper/READ_CTRL ==
  In1 : Inport
  In2 : Inport  Port=2
  Constant : Constant  Value=0  OutDataTypeStr=fixdt(0,8,0)  SampleTime=1/fs
  Switch : Switch  Criteria=u2 ~= 0
  Out1 : Outport  VectorParamsAs1DForOutWhenUnconnected=off
  wires:
  Switch/1 -> Out1/1
  In1/1 -> Switch/1
  In2/1 -> Switch/2
  Constant/1 -> Switch/3

== matlab function OFDM_Tx_HW/OFDMTx/DataGenerator/Data Multiplexer ==
  data: symbols input; dataready input; data output; pilots input; pval input; sts input; stsval input; lts input; ltsval input
function data  = dataMux(symbols,dataready,pilots,pval,sts,stsval,lts,ltsval)
% Data multiplexer 
if (pval == true)
    data = pilots; 
elseif (stsval == true)
    data = sts; 
elseif (ltsval == true)
    data = lts; 
elseif (dataready == true) 
    data = symbols;
else 
    data = fi(complex(0),1,16,14);
end

== matlab function OFDM_Tx_HW/OFDMTx/ControlSignalGenerator/Control Signal Generator ==
  data: enable input; preambleValid output; dataValid output; dataReady output; pilotValid output
function [preambleValid, dataValid, dataReady, pilotValid] = controlSignalGenerator(enable)

        % Constants
    PREAMBLE_LENGTH = 320;
    DATAREADY_LENGTH = 80;
    SUB_FRAME_SIZE = 80;
    OFDM_FRAME_SIZE = 127;
    OFDM_TOTAL_SAMPLES = OFDM_FRAME_SIZE * SUB_FRAME_SIZE;
    
    % States
    IDLE = 0;
    PREAMBLE = 1;
    DATA = 2;
    WAIT = 3;
    
    persistent state reg count
    
    if isempty(state)
        state = fi(IDLE,0,3,0);
        reg = struct(...
            'preambleValid',    false,...
            'dataValid',        false,...
            'dataReady',        false,...
            'pilotValid',       false,...
            'enable',           false,...
            'preamble_flag',    false,...
            'frame_flag',       false);
        count = struct(...
            'preamble',     fi(0,0,ceil(log2(PREAMBLE_LENGTH+1)),0),...
            'dataReady',    fi(0,0,ceil(log2(DATAREADY_LENGTH+1)),0),...
            'frame',        fi(0,0,ceil(log2(OFDM_TOTAL_SAMPLES+1)),0));
    end
    
    % Outputs
    pre_valid = false;
    preambleValid = reg.preambleValid;
    dataValid = false;
    dataReady = false;
    pilotValid = false;
    
    if ~enable
        state(:) = IDLE;
    end
    
    switch state
        case IDLE
            if enable && ~reg.enable
                state(:) = PREAMBLE;
            end
        case PREAMBLE
            if enable
                if count.preamble == PREAMBLE_LENGTH
                    count.preamble(:) = 0;
                    pre_valid = false;
                    state(:) = DATA;
                else
                    count.preamble(:) = count.preamble + 1;
                    pre_valid = true;
                end
            else
                count.preamble(:) = 0;
            end            
        case DATA
            % Data Valid Gen
            dataValid = ~reg.preambleValid && reg.enable;
            % Data Ready Gen
            if dataValid
                if count.dataReady > 31
                    dataReady = true;
                end
                
                % Pilot Valid Gen
                if (count.dataReady < 32) && (count.dataReady > 27)
                    pilotValid = true;
                end
                
                if count.dataReady < DATAREADY_LENGTH - 1
                    count.dataReady(:) = count.dataReady + 1;
                else
                    count.dataReady(:) = 0;
                end
            else
                count.dataReady(:) = 0;
            end
            
            if count.frame < OFDM_TOTAL_SAMPLES-1
                count.frame(:) = count.frame + 1;
            else
                count.frame(:) = 0;
                state(:) = WAIT;
            end
            
        case WAIT
            if count.frame < OFDM_TOTAL_SAMPLES-1
                count.frame(:) = count.frame + 1;
            else
                count.frame(:) = 0;
                state(:) = PREAMBLE;
            end
    end

    % Update registers
    reg.enable = enable;
    reg.preambleValid = pre_valid;
end

== matlab function OFDM_Tx_HW/OFDMTx/CPAdd/Mux2 ==
  data: sts input; stsval input; lts input; ltsval input; dataOut output; data input; dataval input
function dataOut = mux(sts,stsval,lts,ltsval,data,dataval)

if (stsval == true)
    dataOut = sts; 
elseif (ltsval == true)
    dataOut = lts; 
elseif (dataval == true) 
    dataOut = data; 
else 
    dataOut = fi(complex(0),1,16,14);
end

== matlab function OFDM_Tx_HW/OFDMTx/SCMapper/Mux2 ==
  data: preamb input; preambVal input; dataOut output; data input; dataVal input
function dataOut = mux(preamb,preambVal,data,dataVal)

if (preambVal == true)
    dataOut = preamb; 
elseif (dataVal == true)
    dataOut = data; 
else 
    dataOut = fi(complex(0),1,16,14);
end
